simulink model "LGRproy"  (R2018a)
settings: Solver=VariableStepAuto  StartTime=0.0  StopTime=5  FixedStep=0.01  RelTol=1e-3
values from neighbouring files (symbols this model uses):
  T = 2.5    [P4OscarAvilaControlDigital.m]    (also in Practica2Oscar.m = 1; practica5.m = 0.02; proyectoAvilaSilva.m = 0.01; proyectoAvilaSilva2.m = 0.01)
settings Model: Creator=Oscar  LastModifiedBy=Oscar

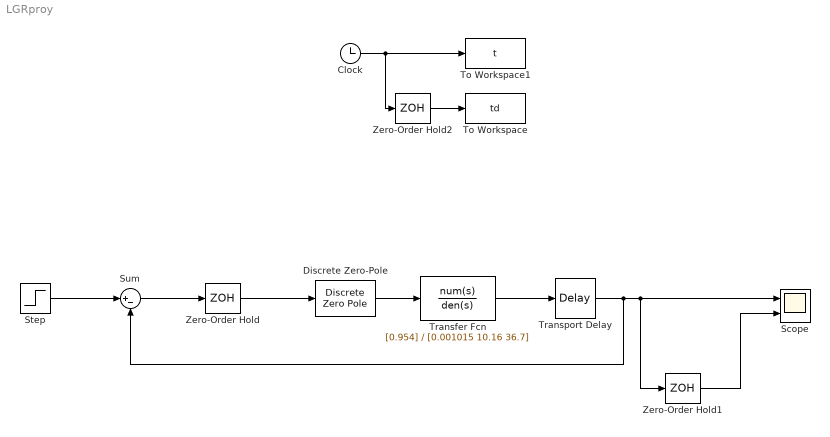
== system LGRproy ==
  Clock : Clock
  Discrete Zero-Pole : DiscreteZeroPole  Zeros=-0.1  Poles=-0.9989  Gain=0.58735  SampleTime=T
  Scope : Scope  NumInputPorts=2
  Step : Step  SampleTime=T
  Sum : Sum  Inputs=|+-
  To Workspace : ToWorkspace  VariableName=td  SampleTime=T
  To Workspace1 : ToWorkspace  VariableName=t  SampleTime=T
  Transfer Fcn : TransferFcn  Numerator=[0.954]  Denominator=[0.001015 10.16 36.7]
  Transport Delay : TransportDelay  DelayTime=0.1
  Zero-Order Hold : ZeroOrderHold  SampleTime=T
  Zero-Order Hold1 : ZeroOrderHold  SampleTime=T
  Zero-Order Hold2 : ZeroOrderHold  SampleTime=T
  wires:
  Zero-Order Hold2/1 -> To Workspace/1
  Clock/1 -> Zero-Order Hold2/1, To Workspace1/1
  Transport Delay/1 -> Sum/2, Zero-Order Hold1/1, Scope/1
  Zero-Order Hold/1 -> Discrete Zero-Pole/1
  Zero-Order Hold1/1 -> Scope/2
  Transfer Fcn/1 -> Transport Delay/1
  Discrete Zero-Pole/1 -> Transfer Fcn/1
  Step/1 -> Sum/1
  Sum/1 -> Zero-Order Hold/1
